simulink model "model_dirigeable"  (R2023b)
settings: Solver=VariableStepAuto  StartTime=0.0  StopTime=25  RelTol=1e-3
settings Model: Creator=ajuton  LastModifiedBy=ajuton

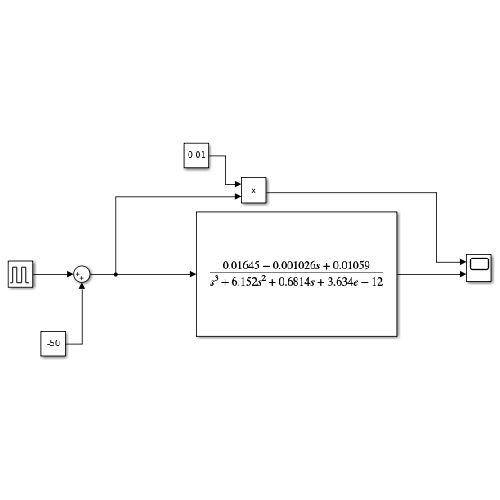
[thumbnail: Simulink's stored preview of the top-level diagram]
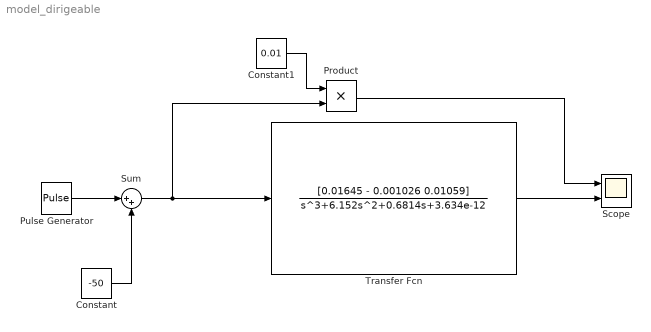
== system model_dirigeable ==
  Constant : Constant  Value=-50
  Constant1 : Constant  Value=0.01
  Product : Product
  Pulse Generator : DiscretePulseGenerator  PulseType=Time based  Amplitude=100  Period=24.6  PulseWidth=33
  Scope : Scope  NumInputPorts=2
  Sum : Sum  Inputs=|++
  Transfer Fcn : TransferFcn  Numerator=[0.01645 - 0.001026 0.01059]  Denominator=[1 6.152 0.6814 3.634e-12]
  wires:
  Pulse Generator/1 -> Sum/1
  Sum/1 -> Product/2, Transfer Fcn/1
  Constant/1 -> Sum/2
  Transfer Fcn/1 -> Scope/2
  Product/1 -> Scope/1
  Constant1/1 -> Product/1
